simulink model "primer_modelo"  (R2023b)
settings: Solver=VariableStepAuto  StartTime=0.0  StopTime=50  RelTol=1e-3
undefined symbols (not defined in the file or in its folder): m, n
libraries: simulink x2
settings Model: Creator=anruk  LastModifiedBy=anruk

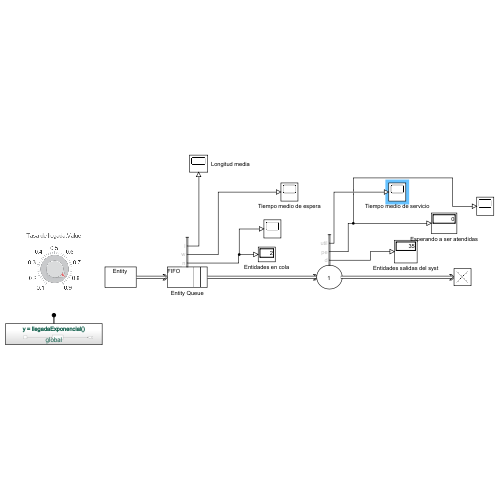
[thumbnail: Simulink's stored preview of the top-level diagram]
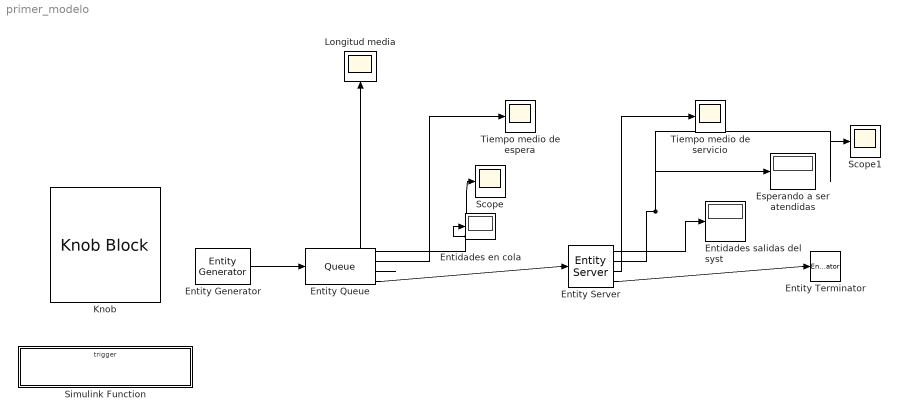
== system primer_modelo ==
  Entidades en cola : Display
  Entidades salidas del syst : Display
  Entity Generator : EntityGenerator  OutputPortMessageModes=m  TimeSource=MATLAB action  IntergenerationTimeAction=dt = llegadaExponencial();  EntityType=Structured  EntityTypeName=Entity
  Entity Queue : Queue  InputPortMessageModes=m  OutputPortMessageModes=n,n,n,m  Capacity=Inf  NumberEntitiesInBlock=on  AverageWait=on  AverageQueueLength=on
      settings: OutputPortMap=o1,o2,o3,o5
  Entity Server : EntityServer  InputPortMessageModes=m  OutputPortMessageModes=n,n,n,m  Capacity=1  ServiceTimeSource=MATLAB action  ServiceTimeAction=|  NumberEntitiesDeparted=on  PendingEntityPresentInBlock=on  Utilization=on
      | % Tiempo de servicio exponencial con tasa de llegada igual a 1
      | media = 1;
      | dt = -media*log(1-rand());
      settings: OutputPortMap=o0,o2,o5,o9
  Entity Terminator : EntityTerminator  InputPortMessageModes=m
  Esperando a ser atendidas : Display
  Knob : KnobBlock  ScaleMin=0.1  ScaleMax=0.9
  Longitud media : Scope
  Scope : Scope
  Scope1 : Scope
  Simulink Function : Subsystem  TreatAsAtomicUnit=on
  Tiempo medio de espera : Scope
  Tiempo medio de servicio : Scope
  wires:
  Entity Generator/1 -> Entity Queue/1
  Entity Queue/4 -> Entity Server/1
  Entity Server/4 -> Entity Terminator/1
  Entity Queue/3 -> Longitud media/1
  Entity Queue/2 -> Tiempo medio de espera/1
  Entity Server/3 -> Tiempo medio de servicio/1
  Entity Server/1 -> Entidades salidas del syst/1
  Entity Queue/1 -> Scope/1, Entidades en cola/1
  Entity Server/2 -> Esperando a ser atendidas/1, Scope1/1

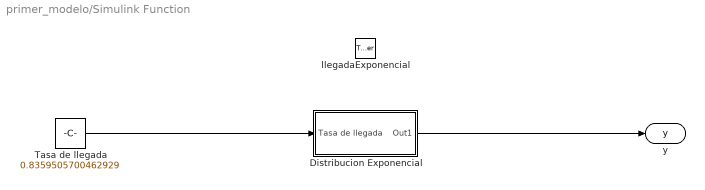
== system primer_modelo/Simulink Function ==
  llegadaExponencial : TriggerPort  TriggerType=function-call  IsSimulinkFunction=on  FunctionName=llegadaExponencial  VariantControl=(inherit)
  Distribucion Exponencial : Subsystem  TreatAsAtomicUnit=on
  Tasa de llegada : Constant  Value=0.8359505700462929
  y : ArgOut  DisableCoverage=on  ArgumentName=y
  wires:
  Tasa de llegada/1 -> Distribucion Exponencial/1(Tasa de llegada)
  Distribucion Exponencial/1(Out1) -> y/1

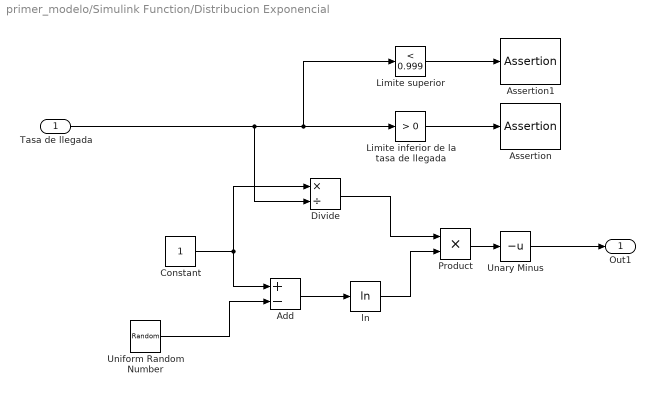
== system primer_modelo/Simulink Function/Distribucion Exponencial ==
  Tasa de llegada : Inport
  Add : Sum  Inputs=+-
  Assertion : Assertion
  Assertion1 : Assertion
  Constant : Constant
  Divide : Product  Inputs=*/
  Limite inferior de la tasa de llegada : simulink/Logic and Bit Operations/Compare To Constant  relop=>  const=0  OutDataTypeStr=boolean
  Limite superior : simulink/Logic and Bit Operations/Compare To Constant  relop=<  const=0.999  OutDataTypeStr=boolean
  Product : Product
  Unary Minus : UnaryMinus
  Uniform Random Number : UniformRandomNumber  Minimum=0  Seed=12345
  ln : Math  Operator=log
  Out1 : Outport
  wires:
  Add/1 -> ln/1
  Uniform Random Number/1 -> Add/2
  Constant/1 -> Divide/1, Add/1
  Limite superior/1 -> Assertion1/1
  Tasa de llegada/1 -> Divide/2, Limite superior/1, Limite inferior de la tasa de llegada/1
  ln/1 -> Product/2
  Divide/1 -> Product/1
  Product/1 -> Unary Minus/1
  Limite inferior de la tasa de llegada/1 -> Assertion/1
  Unary Minus/1 -> Out1/1
